simulink model "chap14_1sim"  (Simulink 8.3)
settings: Solver=ode45  SolverMode=SingleTasking  StartTime=0.0  StopTime=10  FixedStep=0.001  RelTol=1e-3
settings Model: Creator=ljk  LastModifiedBy=Administrator  ExtModeTrigMode=oneshot  ExtModeArmWhenConnect=off
settings DataIOCC: LimitDataPoints=off  SignalLoggingName=sigsOut
settings OptimizationCC: BooleanDataType=off  ExpressionDepthLimit=2147483647
settings DebuggingCC: SaveWithParameterizedLinksMsg=none  SignalResolutionControl=TryResolveAllWithWarning  SolverPrmCheckMsg=none  MultiTaskDSMMsg=warning  MultiTaskCondExecSysMsg=none  FcnCallInpInsideContextMsg=EnableAllAsWarning
settings HardwareCC: TargetUnknown=on
settings RTWCC: IncludeERTFirstTime=on

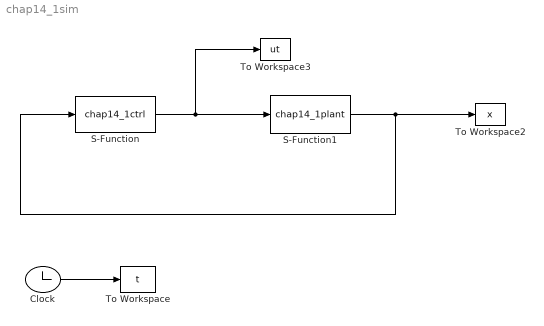
== system chap14_1sim ==
  Clock : Clock
  S-Function : S-Function  FunctionName=chap14_1ctrl  EnableBusSupport=off
  S-Function1 : S-Function  FunctionName=chap14_1plant  EnableBusSupport=off
  To Workspace : ToWorkspace  VariableName=t  SampleTime=-1
  To Workspace2 : ToWorkspace  VariableName=x  SampleTime=-1
  To Workspace3 : ToWorkspace  VariableName=ut  SampleTime=-1
  wires:
  Clock/1 -> To Workspace/1
  S-Function1/1 -> To Workspace2/1, S-Function/1
  S-Function/1 -> S-Function1/1, To Workspace3/1
